simulink model "chapt5_MPC_Dynamics"  (Simulink 8.2)
settings: Solver=ode45  StartTime=0.0  StopTime=40  FixedStep=0.01  RelTol=1e-3
libraries: Solver_SF x1, simulink x1
settings Model: Creator=xuwei  LastModifiedBy=liuho
settings ConfigurationSet: Description=SimMechanics 2G

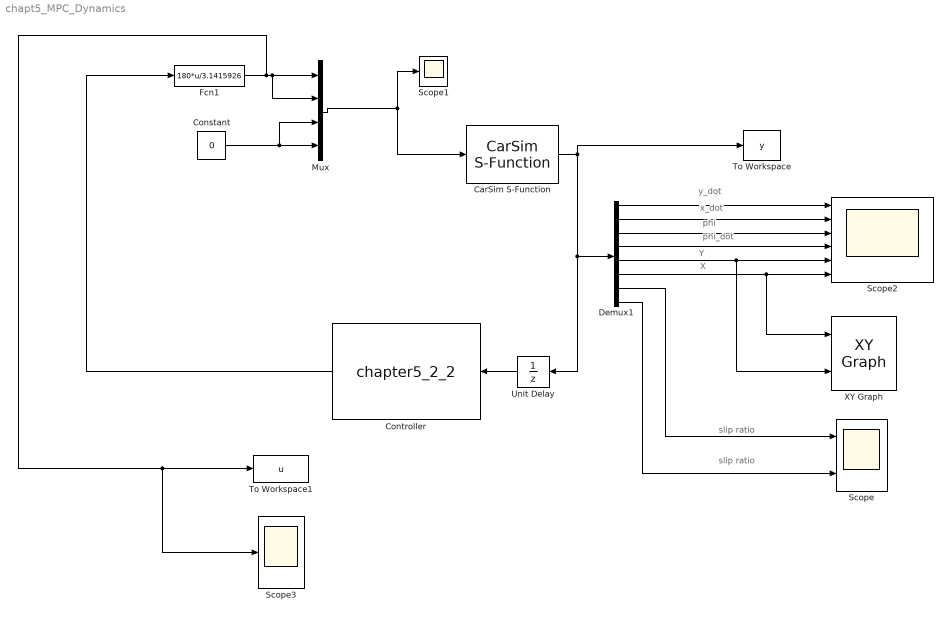
== system chapt5_MPC_Dynamics ==
  note: y_dot
  note: x_dot
  note: phi
  note: phi_dot
  note: Y
  note: X
  note: slip ratio
  note: slip ratio
  CarSim S-Function : Solver_SF/CarSim S-Function  Priority=1  VehicleCode=i_i  SIMFILE=simfile.sim
  Constant : Constant  Value=0
  Controller : S-Function  FunctionName=chapter5_2_2  EnableBusSupport=off
  Demux1 : Demux  Outputs=8
  Fcn1 : Fcn  Expr=180*u/3.1415926
  Mux : Mux
  Scope : Scope  NumInputPorts=2
      settings: YMin=-5~-5  YMax=5~5
  Scope1 : Scope
      settings: SaveName=ScopeData2
  Scope2 : Scope  NumInputPorts=6
      settings: TimeRange=20  YMin=-1~35~-10~-20~-4~0  YMax=1~36.5~5~20~2~200
  Scope3 : Scope
      settings: SaveName=ScopeData3
  To Workspace : ToWorkspace  VariableName=y  SampleTime=-1  SaveFormat=Structure
  To Workspace1 : ToWorkspace  VariableName=u  SampleTime=-1  SaveFormat=Structure
  Unit Delay : UnitDelay  SampleTime=-1
  XY Graph : simulink/Sinks/XY Graph  xmin=0  xmax=200  ymin=-2  ymax=4  st=-1
  wires:
  CarSim S-Function/1 -> Unit Delay/1, Demux1/1, To Workspace/1
  Demux1/1 -> Scope2/1
  Demux1/2 -> Scope2/2
  Demux1/3 -> Scope2/3
  Demux1/4 -> Scope2/4
  Demux1/5 -> XY Graph/2, Scope2/5
  Demux1/6 -> XY Graph/1, Scope2/6
  Unit Delay/1 -> Controller/1
  Demux1/7 -> Scope/1
  Demux1/8 -> Scope/2
  Mux/1 -> CarSim S-Function/1, Scope1/1
  Controller/1 -> Fcn1/1
  Constant/1 -> Mux/3, Mux/4
  Fcn1/1 -> Scope3/1, To Workspace1/1, Mux/2, Mux/1
